simulink model "Power_Model_Official_Pars"  (R2023a)
settings: Solver=ode23t  StartTime=0.0  StopTime=1000  FixedStep=0.01  MaxStep=0.01  RelTol=1e-3  AbsTol=1e-3
values from neighbouring files (symbols this model uses):
  anode_tube_D = 0.01    [fuel_cell_battery_par.mat]
  cathode_tube_D = 0.05    [fuel_cell_battery_par.mat]
  comp_rpm_TLU = [0 1800 3600]    [fuel_cell_battery_par.mat]
  coolant_num_layers = 20    [fuel_cell_battery_par.mat]
  coolant_num_passes = 12    [fuel_cell_battery_par.mat]
  coolant_tube_D = 0.05    [fuel_cell_battery_par.mat]
  coolant_w_channels = 1    [fuel_cell_battery_par.mat]
  env_p = 0.101325    [fuel_cell_battery_par.mat]
  env_T = 20    [fuel_cell_battery_par.mat]
  env_yH20 = 0.0115436377169    [fuel_cell_battery_par.mat]
  env_yO2 = 0.21    [fuel_cell_battery_par.mat]
  radiator_air_area_fins = 11.5625    [fuel_cell_battery_par.mat]
  radiator_air_area_primary = 1.223125    [fuel_cell_battery_par.mat]
  radiator_eta_fin = 0.7    [fuel_cell_battery_par.mat]
  radiator_N_tubes = 25    [fuel_cell_battery_par.mat]
  radiator_rho = 2700    [fuel_cell_battery_par.mat]
  radiator_t_wall = 0.0001    [fuel_cell_battery_par.mat]
  radiator_tube_H = 0.0015    [fuel_cell_battery_par.mat]
  radiator_W = 0.025    [fuel_cell_battery_par.mat]
  stack_area = 280    [fuel_cell_battery_par.mat]
  stack_iL = 1.4    [fuel_cell_battery_par.mat]
  stack_mea_rho = 1800    [fuel_cell_battery_par.mat]
  stack_num_cells = 400    [fuel_cell_battery_par.mat]
  stack_num_channels = 8    [fuel_cell_battery_par.mat]
  stack_t_gdl = 250    [fuel_cell_battery_par.mat]
  stack_t_membrane = 125    [fuel_cell_battery_par.mat]
  stack_w_channels = 1    [fuel_cell_battery_par.mat]
undefined symbols (not defined in the file or in its folder): Bat, f_fc_auxpower, f_fc_currcmd_bpt, f_fc_h2flow, f_fc_heatflow, f_fc_tmpcmd_bpt, f_fc_voltage, Mot, N2_T
libraries: fl_lib x170, nesl_utility x78, FuelCell_lib x32, simulink x5, slpidlib x4, ee_lib x3, autolibshared x1, batteryecm_lib x1, simulink_extras x1
(part 1 of 9)
settings Model: Creator=Learning  LastModifiedBy=Leviathan
settings SolverCC: ZeroCrossAlgorithm=Adaptive
settings OptimizationCC: ReuseModelBlockBuffer=off
settings DebuggingCC: IgnoredZcDiagnostic=none
settings ModelReferenceCC: EnableRefExpFcnMdlSchedulingChecks=on
settings SimscapeCC: SimscapeLogType=all  SimscapeLogSimulationStatistics=on  SimscapeLogLimitData=off

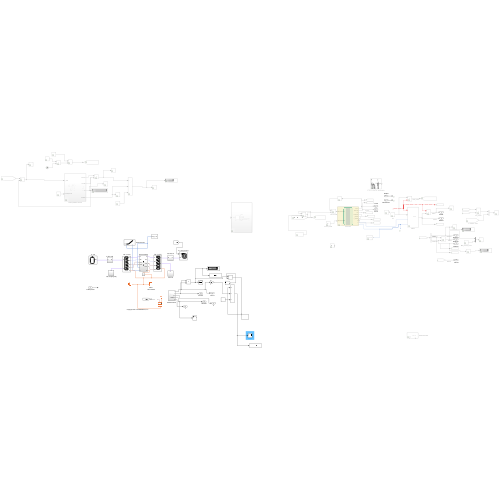
[thumbnail: Simulink's stored preview of the top-level diagram]
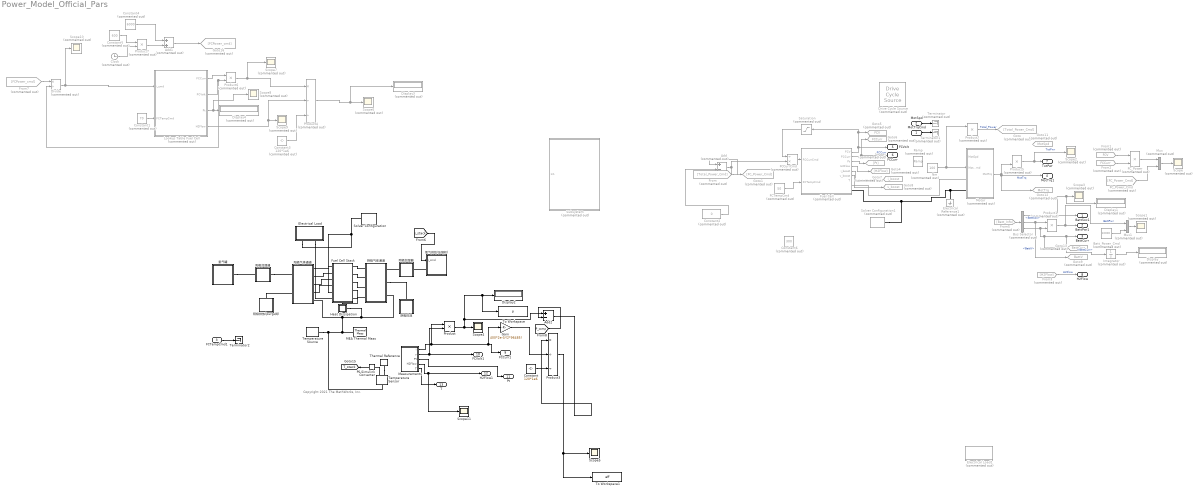
== system Power_Model_Official_Pars ==
  note: Copyright 2021 The MathWorks, Inc.
  MotTrqCmd : Inport
  MotSpd : Inport  Port=2
  FCTempCmd1 : Inport  Port=3
  Add : Sum  Commented=on  Inputs=+-
  Add1 : Sum  Commented=on
  Add2 : Sum  Inputs=+-
  Batt_Power_Cmd : Constant  Commented=on  Value=10000
  Bus Selector : BusSelector  Commented=on  OutputSignals=BattSoc,BattV,BattCurr
  Clock : Clock  Commented=on
  Constant : Constant  Value=120*1e6
  Constant1 : Constant  Commented=on  Value=70
  Constant2 : Constant  Commented=on  Value=0
  Constant3 : Constant  Commented=on  Value=120*1e6
  Constant4 : Constant  Commented=on  Value=6000
  Constant5 : Constant  Commented=on  Value=600
  Constant6 : Constant  Commented=on  Value=300
  Display{,1,3..4} (4 alike) : Display  Commented=on
  Display2 : Display
  Divide : Product  Commented=on  Inputs=*/
  Drive Cycle Source : autolibshared/Drive Cycle Source  Commented=on  cycleVar=FTP75  fileVar=L:\Bauto\matlab\test\toolbox\shared\autoblks\scenario\adac.txt  tfinal="2474  seconds"  cycleRepeat=off  outAccPort=off  outGearPort=off  gearList=No gear data  t_wot1=1  xdot_woto=0  xdot_wot1=26.8  t_wot2=30  xdot_wot2=0  t_wotend=40  srcUnit=m/s  outUnit=m/s  srcAccUnit=m/s/s  outAccUnit=m/s^2  dt=0  aMode=1  faultOption=off  velBnd=2  velBndUnit=mph  inUnit=m/s  timeBnd=1  failOption=off  stopSim=off  maxFaultCnt=10  maxFaultTime=2  maxTotFaultTime=15  traceOption=off  dtTrace=1  traceWindow=10  lastDCname=FTP75  lastOutUnit=mph  lastDT=0  lastTB=1  lastSB=2  forceCalcBound=off
  Electrical Load : Subsystem  Tag=PublishSubsystem  mask(Electrical Load){input_type=Ramp}
      mask prompts: input_type "Select one of the following scenarios:"
      settings: PortSchema="{\"entries\":[{\"content\":{\"sides\":[{\"content\":{},\"type\":\"ConnectorPlacement.EquallySpacedRectSide\",\"uuid\":\"cf26c57a-4aaa-4eca-a1cf-dab3379228b7\"},{\"content\":{\"side\":\"RIGHT\"},\"type\":\"ConnectorPlacement.EquallySpacedRectSide\",\"uuid\":\"bd4a28c6-f8d3-4492-9f61-a12eb17ccdd3\"},{\"content\":{\"side\":\"TOP\"},\"type\":\"ConnectorPlacement.EquallySpacedRectSide\",\"uuid\":\"7f54a4db-ccf4-4e3a-a135-4ada067d241f\"},{\"content\":{\"connectorIds\":[\"RConn1\",\"RConn2\"],\"side\":\"BOTTOM\"},\"type\":\"ConnectorPlacement.EquallySpacedRectSide\",\"uuid\":\"8817983d-3f79-43b3-9594-6d12f7dcf066\"}]},\"type\":\"ConnectorPlacement.EquallySpacedConnector\",\"uuid\":\"79253ea6-cd7f-4983-840a-f5cee3a4dd91\"}],\"packageUris\":[\"http://schema.mathworks.com/mf0/Connector/R2020b\"],\"version\":\"1.0\"}"
      mask TypeOptions input_type: Drive cycle | Ramp | Step
      mask Callback input_type:
      | activeVariant = get_param(gcb, 'input_type');
      | set_param([gcb '/Inputs'], 'OverrideUsingVariant', activeVariant)
      mask Display:
      | blk = get_param([gcb, '/Inputs'], 'CompiledActiveChoiceBlock');
      | eval(get_param(blk, 'MaskDisplay'))
  Electrical Load1 : Subsystem  Tag=PublishSubsystem  Commented=on  mask(Electrical Load){input_type=Ramp}
      mask prompts: input_type "Select one of the following scenarios:"
      settings: PortSchema="{\"entries\":[{\"content\":{\"sides\":[{\"content\":{},\"type\":\"ConnectorPlacement.EquallySpacedRectSide\",\"uuid\":\"cf26c57a-4aaa-4eca-a1cf-dab3379228b7\"},{\"content\":{\"side\":\"RIGHT\"},\"type\":\"ConnectorPlacement.EquallySpacedRectSide\",\"uuid\":\"bd4a28c6-f8d3-4492-9f61-a12eb17ccdd3\"},{\"content\":{\"side\":\"TOP\"},\"type\":\"ConnectorPlacement.EquallySpacedRectSide\",\"uuid\":\"7f54a4db-ccf4-4e3a-a135-4ada067d241f\"},{\"content\":{\"connectorIds\":[\"RConn1\",\"RConn2\"],\"side\":\"BOTTOM\"},\"type\":\"ConnectorPlacement.EquallySpacedRectSide\",\"uuid\":\"8817983d-3f79-43b3-9594-6d12f7dcf066\"}]},\"type\":\"ConnectorPlacement.EquallySpacedConnector\",\"uuid\":\"79253ea6-cd7f-4983-840a-f5cee3a4dd91\"}],\"packageUris\":[\"http://schema.mathworks.com/mf0/Connector/R2020b\"],\"version\":\"1.0\"}"
      mask TypeOptions input_type: Drive cycle | Ramp | Step
      mask Callback input_type:
      | activeVariant = get_param(gcb, 'input_type');
      | set_param([gcb '/Inputs'], 'OverrideUsingVariant', activeVariant)
      mask Display:
      | blk = get_param([gcb, '/Inputs'], 'CompiledActiveChoiceBlock');
      | eval(get_param(blk, 'MaskDisplay'))
  Electrical Reference1 : fl_lib/Electrical/Electrical Elements/Electrical Reference  Commented=on
  FCCurrCmd : Product  Commented=on  Inputs=/*
  FCTempCmd : Constant  Commented=on  Value=50
  FC_Power : Product  Commented=on
  FC_Power_Cmd : From  Commented=on  GotoTag=FC_Power_Cmd
  From : From  Commented=on  GotoTag=Total_Power_Cmd
  From1 : From  Commented=on  GotoTag=FCV  TagVisibility=global
  From2 : From  Commented=on  GotoTag=FCCurr  TagVisibility=global
  From3 : From  Commented=on  GotoTag=H2Flow
  From5 : From  Commented=on  GotoTag=Batt_Info
  From7 : From  Commented=on  GotoTag=FCPower_cmd
  Fuel Cell : Subsystem  Commented=on  VariantControl=0
      mask Display: image('fuel_cell_converter_IMAGE.png'); % Use "Edit Image" on toolstrip to change.
  Fuel Cell Stack : Subsystem  VariantControl=SSC
  Gain : Gain  Gain=400*2e-3/(2*96485)
  Goto : Goto  Commented=on  GotoTag=Total_Power_Cmd
  Goto1 : Goto  Commented=on  GotoTag=FC_Power_Cmd
  Goto11 : Goto  Commented=on  GotoTag=MotSpd  TagVisibility=global
  Goto12 : Goto  Commented=on  GotoTag=MotTrq  TagVisibility=global
  Goto13 : Goto  Commented=on  GotoTag=BattCurr  TagVisibility=global
  Goto16 : Goto  Commented=on  GotoTag=FCPower_cmd
  Goto2 : Goto  Commented=on  GotoTag=Pt
  Goto4 : Goto  Commented=on  GotoTag=H2Flow
  Goto5 : Goto  Commented=on  GotoTag=FCV  TagVisibility=global
  Goto6 : Goto  Commented=on  GotoTag=FCCurr  TagVisibility=global
  Goto7 : Goto  Commented=on  GotoTag=i_boost  TagVisibility=global
  Goto8 : Goto  Commented=on  GotoTag=v_boost  TagVisibility=global
  Goto9 : Goto  Commented=on  GotoTag=BattV  TagVisibility=global
  Heat Dissipation : Subsystem
      settings: PortSchema="{\"entries\":[{\"content\":{\"sides\":[{\"content\":{},\"type\":\"ConnectorPlacement.EquallySpacedRectSide\",\"uuid\":\"40b2385a-b20e-464f-8016-3228e4acac4a\"},{\"content\":{\"connectorIds\":[\"RConn1\"],\"side\":\"RIGHT\"},\"type\":\"ConnectorPlacement.EquallySpacedRectSide\",\"uuid\":\"0e95dc4b-d2da-4ab6-a6e9-e2cb275776ce\"},{\"content\":{\"connectorIds\":[\"LConn1\"],\"side\":\"TOP\"},\"type\":\"ConnectorPlacement.EquallySpacedRectSide\",\"uuid\":\"0f5995c7-26f6-433d-889b-dea78bcd2b2a\"},{\"content\":{\"side\":\"BOTTOM\"},\"type\":\"ConnectorPlacement.EquallySpacedRectSide\",\"uuid\":\"a2ee1c19-f9e9-4dbd-a9ff-92feea387e85\"}]},\"type\":\"ConnectorPlacement.EquallySpacedConnector\",\"uuid\":\"721753ea-9ada-4c74-8c6f-50b905d96904\"}],\"packageUris\":[\"http://schema.mathworks.com/mf0/Connector/R2020b\"],\"version\":\"1.0\"}"
  Integrator : Integrator  Commented=on
  Lookup Table Fuel Cell : Subsystem  Commented=on  VariantControl=Choice_3
      settings: PortSchema="{\"entries\":[{\"content\":{\"sides\":[{\"content\":{},\"type\":\"ConnectorPlacement.EquallySpacedRectSide\",\"uuid\":\"32248e1c-8adb-4301-a735-652c844f38d9\"},{\"content\":{\"side\":\"RIGHT\"},\"type\":\"ConnectorPlacement.EquallySpacedRectSide\",\"uuid\":\"e199895e-2a46-4791-8ec6-c72fbddb281a\"},{\"content\":{\"connectorIds\":[\"In1\",\"In2\"],\"side\":\"TOP\"},\"type\":\"ConnectorPlacement.EquallySpacedRectSide\",\"uuid\":\"d27f5cfc-8d50-4a08-b63d-60966cdd3a3e\"},{\"content\":{\"connectorIds\":[\"Out1\",\"Out2\",\"Out3\",\"Out4\"],\"side\":\"BOTTOM\"},\"type\":\"ConnectorPlacement.EquallySpacedRectSide\",\"uuid\":\"4de9f516-5cfd-4c93-92a2-161937995774\"}]},\"type\":\"ConnectorPlacement.EquallySpacedConnector\",\"uuid\":\"ebb74780-6fd4-4e24-9636-290cc1e1e603\"}],\"packageUris\":[\"http://schema.mathworks.com/mf0/Connector/R2020b\"],\"version\":\"1.0\"}"
  MEA Thermal Mass : fl_lib/Thermal/Thermal Elements/Thermal Mass  mass_type=foundation.enum.constant_variable.constant  mass=stack_mea_rho * stack_area*1e-4 * (stack_t_membrane + 2*stack_t_gdl)*1e-6 * stack_num_cells kg  sp_heat=stack_mea_cp J/kg/K  mass_min=1e-6 kg  num_ports=foundation.enum.numPorts2.one  m_specify=off  m_priority=High  m=1 kg  m_nominal_specify=off  m_nominal_unit=kg  m_nominal_value=1  T_specify=on  T_priority=High  T=env_T degC  T_nominal_specify=off  T_nominal_unit=K  T_nominal_value=1  Q_specify=off  Q_priority=None  Q=0 W  Q_nominal_specify=off  Q_nominal_unit=W  Q_nominal_value=1
  Measurements : Subsystem
  Motor : Subsystem  Commented=on
      mask Display: image('E:\Graduation Project File\Fuel_cell\Fuel_cell_model\Model_figure\emotor_simplified_IMAGE.png'); % 使用工具条上的 "编辑图像" 进行更改。
  Mux : Mux  Commented=on  Inputs=2
  Mux1 : Mux  Commented=on  Inputs=2
  Nm : Constant  Commented=on  Value=100
  PS-Simulink Converter : nesl_utility/PS-Simulink Converter  PhysicalDomain=network_engine_domain  SubClassName=ps_output  LeftPortType=input  RightPortType=output  PseudoPeriodic=off  Frequencies=[]  VectorFormat=1-D array  Unit=degC  AffineConversion=on
  Product : Product
  Product{1..2,5..7} (5 alike) : Product  Commented=on
  Product3 : Product  Inputs=*//
  Product4 : Product  Commented=on  Inputs=*//
  Ramp : simulink/Sources/Ramp  Commented=on  slope=1  start=0  InitialOutput=0
  Saturation : Saturate  Commented=on  UpperLimit=inf  LowerLimit=250
  Scope{,1..3,6..10} (9 alike) : Scope  Commented=on
  Scope11 : Scope
  Scope4 : Scope
  Scope5 : Scope
  Solver Configuration : nesl_utility/Solver Configuration  PhysicalDomain=network_engine_domain  SubClassName=solver  LeftPortType=input  RightPortType=generic  Tones=[]  Harmonics=[]  SimulateNoise=off  Profile=off  UseLocalSampling=off  EnableSwitchedLinearOptims=on  FrequencyDomain=off  UseCCode=off  RelTol=0.001  AbsTol=1e-06  MinStep=1e-09  ToWorkspace=off  RevertToSquareIcSolve=off  NumHomotopyIterations=100  PhasorMode=off  PhasorModeNumHarmonics=1  ConsistencySolver=NEWTON_XTOL_AFTER_FTOL  IndexReductionMethod=DerivativeReplacement  DoDC=off  ResidualTolerance=1e-09  ConsistencyTolSource=GLOBAL  ConsistencyAbsTol=0.001  ConsistencyRelTol=0.001  ConsistencyTolFactor=0.001  UseLocalSolver=off  LocalSolverChoice=NE_BACKWARD_EULER_ADVANCER  ResolveIndetEquations=on  FunctionEvalNumThread=1  LocalSolverSampleTime=0.001  DoFixedCost=off  MaxNonlinIter=3  MaxModeIter=2  ComputeImpulses=off  ImpulseIterations=2  LinearAlgebra=auto  LinearAlgebraNumThread=0  EquationFormulation=NE_TIME_EF  DelaysMemoryBudget=1024  AutomaticFiltering=on  FilteringTimeConstant=0.001  PartitionStorageMethod=AS_NEEDED  PartitionMemoryBudget=1024  PartitionMethod=ROBUST
  Solver Configuration1 : nesl_utility/Solver Configuration  Commented=on  PhysicalDomain=network_engine_domain  SubClassName=solver  LeftPortType=input  RightPortType=generic  Tones=[]  Harmonics=[]  SimulateNoise=off  Profile=off  UseLocalSampling=off  EnableSwitchedLinearOptims=on  FrequencyDomain=off  UseCCode=off  RelTol=0.001  AbsTol=1e-06  MinStep=1e-09  ToWorkspace=off  RevertToSquareIcSolve=off  NumHomotopyIterations=100  PhasorMode=off  PhasorModeNumHarmonics=1  ConsistencySolver=NEWTON_XTOL_AFTER_FTOL  IndexReductionMethod=DerivativeReplacement  DoDC=off  ResidualTolerance=1e-09  ConsistencyTolSource=GLOBAL  ConsistencyAbsTol=0.001  ConsistencyRelTol=0.001  ConsistencyTolFactor=0.001  UseLocalSolver=off  LocalSolverChoice=NE_BACKWARD_EULER_ADVANCER  ResolveIndetEquations=on  FunctionEvalNumThread=1  LocalSolverSampleTime=0.001  DoFixedCost=off  MaxNonlinIter=3  MaxModeIter=2  ComputeImpulses=off  ImpulseIterations=2  LinearAlgebra=auto  LinearAlgebraNumThread=0  EquationFormulation=NE_TIME_EF  DelaysMemoryBudget=1024  AutomaticFiltering=on  FilteringTimeConstant=0.001  PartitionStorageMethod=AS_NEEDED  PartitionMemoryBudget=1024  PartitionMethod=ROBUST
  Subsystem : Subsystem  Commented=on
  Temperature Sensor : fl_lib/Thermal/Thermal Sensors/Temperature Sensor  temperature_measure=foundation.enum.MeasurementReference.difference
  Temperature Source : fl_lib/Thermal/Thermal Sources/Temperature Source  temperature=70 degC
  Terminator : Terminator  Commented=on
  Terminator1 : Terminator  Commented=on
  Terminator2 : Terminator
  Thermal Reference : fl_lib/Thermal/Thermal Elements/Thermal Reference
  To Workspace : ToWorkspace  VariableName=p  SampleTime=1
  To Workspace1 : ToWorkspace  VariableName=eff  SampleTime=1
  氢气罐 : Subsystem  Tag=PublishSubsystem
      mask Display:
      | plot(0, 0)
      | plot(100, 100)
      | 
      | n = 20;
      | r = 20;
      | x1 = 15;
      | x2 = 65;
      | y1 = 5;
      | y2 = 85;
      | 
      | plot([x1 x1], [y1+r y2-r])
      | plot([x1+r x2-r], [y2 y2])
      | plot([x2 x2], [y2-r y1+r])
      | plot([x2-r x1+r], [y1 y1])
      | 
      | plot(cos(linspace(pi/2, pi, n))*r + x1+r, sin(linspace(pi/2, pi, n))*r + y2-r)
      | plot(cos(linspace(0, pi/2, n))*r + x2-r, sin(linspace(0, pi/2, n))*r + y2-r)
      | plot(cos(linspace(3*pi/2, 2*pi, n))*r + x2-r, sin(linspace(3*pi/2, 2*pi, n))*r + y1+r)
      | plot(cos(linspace(pi, 3*pi/2, n))*r + x1+r, sin(linspace(pi, 3*pi/2, n))*r + y1+r)
      | 
      | plot([-5 -5 5 5] + (x1+x2)/2, [0 5 5 0] + y2)
  氧气供给(压缩机) : Subsystem  Tag=PublishSubsystem
      mask Display:
      | plot(0, 0)
      | plot(100, 100)
      | 
      | n = 80;
      | r1 = 15;
      | r2 = 30;
      | 
      | plot(cos(linspace(0, 2*pi, n))*r1 + 65, sin(linspace(0, 2*pi, n))*r1 + 50)
      | plot(cos(linspace(0, 2*pi, n))*r2 + 65, sin(linspace(0, 2*pi, n))*r2 + 50)
      | 
      | plot([65 30 30 42], [80 80 70 70])
  阳极加湿器 : Subsystem  Tag=PublishSubsystem
  阳极排放(purge阀) : Subsystem  Tag=PublishSubsystem
      settings: PortSchema="{\"entries\":[{\"content\":{\"sides\":[{\"content\":{\"connectorIds\":[]},\"type\":\"ConnectorPlacement.EquallySpacedRectSide\",\"uuid\":\"6344d1cf-22ea-4a51-9588-07afca0fac15\"},{\"content\":{\"connectorIds\":[],\"side\":\"RIGHT\"},\"type\":\"ConnectorPlacement.EquallySpacedRectSide\",\"uuid\":\"a3908f81-9410-4056-87cd-9faba76d3fb8\"},{\"content\":{\"connectorIds\":[\"LConn1\"],\"side\":\"TOP\"},\"type\":\"ConnectorPlacement.EquallySpacedRectSide\",\"uuid\":\"a1c9e24d-adb9-4361-8e9b-feafccbbdb81\"}]},\"type\":\"ConnectorPlacement.EquallySpacedConnector\",\"uuid\":\"d5180d8f-18a0-491d-9fff-909db43c9aea\"}],\"packageUris\":[\"http://schema.mathworks.com/mf0/Connector/R2020b\"],\"version\":\"1.0\"}"
  阳极气体通道 : Subsystem  Tag=PublishSubsystem
      mask Display:
      | plot(0, 0)
      | plot(100, 100)
      | 
      | x1 = 25;
      | x2 = 65;
      | y1 = 23;
      | y2 = 95;
      | xt = 15;
      | yt = 9;
      | 
      | x_pattern = [x2 x2    x1+xt x1+xt   x1+xt   x2     ];
      | y_pattern = [y2 y2-yt y2-yt y2-2*yt y2-2*yt y2-2*yt];
      | 
      | plot([x1 x1 x2 x_pattern x_pattern      x_pattern      x_pattern         x2    x1], ...
      |      [y1-yt y2 y2 y_pattern y_pattern-2*yt y_pattern-4*yt y_pattern-6*yt y1-yt y1-yt])
  阴极加湿器 : Subsystem  Tag=PublishSubsystem
  阴极排放 : Subsystem  Tag=PublishSubsystem
      settings: PortSchema="{\"entries\":[{\"content\":{\"sides\":[{\"content\":{\"connectorIds\":[]},\"type\":\"ConnectorPlacement.EquallySpacedRectSide\",\"uuid\":\"6344d1cf-22ea-4a51-9588-07afca0fac15\"},{\"content\":{\"connectorIds\":[],\"side\":\"RIGHT\"},\"type\":\"ConnectorPlacement.EquallySpacedRectSide\",\"uuid\":\"a3908f81-9410-4056-87cd-9faba76d3fb8\"},{\"content\":{\"connectorIds\":[\"LConn1\"],\"side\":\"TOP\"},\"type\":\"ConnectorPlacement.EquallySpacedRectSide\",\"uuid\":\"a1c9e24d-adb9-4361-8e9b-feafccbbdb81\"}]},\"type\":\"ConnectorPlacement.EquallySpacedConnector\",\"uuid\":\"d5180d8f-18a0-491d-9fff-909db43c9aea\"}],\"packageUris\":[\"http://schema.mathworks.com/mf0/Connector/R2020b\"],\"version\":\"1.0\"}"
  阴极气体通道 : Subsystem  Tag=PublishSubsystem
      mask Display:
      | plot(0, 0)
      | plot(100, 100)
      | 
      | x1 = 35;
      | x2 = 75;
      | y1 = 23;
      | y2 = 95;
      | xt = 15;
      | yt = 9;
      | 
      | x_pattern = [x1 x1    x2-xt x2-xt   x2-xt   x1     ];
      | y_pattern = [y2 y2-yt y2-yt y2-2*yt y2-2*yt y2-2*yt];
      | 
      | plot([x2 x2 x1 x_pattern x_pattern      x_pattern      x_pattern         x1    x2], ...
      |      [y1-yt y2 y2 y_pattern y_pattern-2*yt y_pattern-4*yt y_pattern-6*yt y1-yt y1-yt])
  BattSoc1 : Outport  VectorParamsAs1DForOutWhenUnconnected=off
  BattPwr1 : Outport  Port=2  VectorParamsAs1DForOutWhenUnconnected=off
  BattCurr : Outport  Port=3  VectorParamsAs1DForOutWhenUnconnected=off
  MotTrq1 : Outport  Port=4  VectorParamsAs1DForOutWhenUnconnected=off
  FCVolt : Outport  Port=5  VectorParamsAs1DForOutWhenUnconnected=off
  FCCurr : Outport  Port=6  VectorParamsAs1DForOutWhenUnconnected=off
  TotPwr : Outport  Port=7
  H2Flow : Outport  Port=8  VectorParamsAs1DForOutWhenUnconnected=off
  FCCurr1 : Outport  Port=9
  FCVolt1 : Outport  Port=10
  Pt : Outport  Port=11
  H2Flow1 : Outport  Port=12
  T : Outport  Port=13
  tag scope: T_stack=global
  wires:
  Bus Selector/1 -> Display1/1, Scope3/1, BattSoc1/1  "<BattSoc>"
  FCTempCmd/1 -> Fuel Cell/2(FCTempCmd)
  Motor/1(MotTrq) -> Goto12/1, MotTrq1/1, Product5/2  "MotTrq"
  From3/1 -> H2Flow/1  "H2Flow"
  Product5/1 -> Scope2/1, TotPwr/1  "TotPwr"
  ? -> Product2/2, Product5/1, Goto11/1, Motor/1(MotSpd)
  Bus Selector/3 -> Goto13/1, Integrator/1, BattCurr/1, Product1/2  "<BattCurr>"
  Product1/1 -> Mux1/1, BattPwr1/1  "BattPwr"
  Fuel Cell/5(i_boost) -> Goto7/1
  From5/1 -> Bus Selector/1
  Nm/1 -> Product2/1, Motor/2(MotTrqCmd)
  Fuel Cell/2(FCCurr) -> Goto6/1, FCCurr/1  "FCCurr"
  Fuel Cell/3(Pt) -> Goto2/1
  Bus Selector/2 -> Product1/1, Goto9/1  "<BattV>"
  FCCurrCmd/1 -> Fuel Cell/1(FCCurrCmd)
  Saturation/1 -> FCCurrCmd/1
  MotSpd/1 -> Terminator/1
  MotTrqCmd/1 -> Terminator1/1
  Product2/1 -> Goto/1  "Total_Power"
  From/1 -> Add/1
  Constant2/1 -> Add/2
  Add/1 -> Goto1/1, FCCurrCmd/2
  From1/1 -> FC_Power/1
  From2/1 -> FC_Power/2
  Mux/1 -> Scope/1
  FC_Power/1 -> Mux/1
  FC_Power_Cmd/1 -> Mux/2
  Mux1/1 -> Scope1/1
  Batt_Power_Cmd/1 -> Mux1/2
  Fuel Cell/1(FCV) -> Saturation/1, Goto5/1, FCVolt/1
  Fuel Cell/4(H2Flow) -> Goto4/1
  Fuel Cell/6(v_boost) -> Goto8/1
  Integrator/1 -> Display/1
  Measurements/3(Pt) -> Pt/1
  Measurements/5(T) -> T/1
  FCTempCmd1/1 -> Terminator2/1
  PS-Simulink Converter/1 -> [T_stack]
  Measurements/4(H2Flow) -> Scope11/1, H2Flow1/1
  Measurements/1(i) -> Product/1, Gain/1, FCCurr1/1
  Measurements/2(v) -> Product/2, FCVolt1/1
  Product/1 -> Add2/1, To Workspace/1, Display2/1, Scope4/1
  [i_stack] -> 氧气供给(压缩机)/1(i_cmd)
  Constant/1 -> Product3/3
  Product3/1 -> To Workspace1/1, Scope5/1
  Constant1/1 -> Lookup Table Fuel Cell/2(FCTempCmd)
  Lookup Table Fuel Cell/4(H2Flow) -> Product4/2, Scope9/1
  Product4/1 -> Display3/1, Scope6/1
  Constant3/1 -> Product4/3
  Product6/1 -> Scope7/1, Product4/1
  Lookup Table Fuel Cell/1(FCCurr) -> Product6/1
  Lookup Table Fuel Cell/2(FCVolt) -> Divide/2, Product6/2
  From7/1 -> Divide/1
  Clock/1 -> Product7/2
  Constant5/1 -> Product7/1
  Product7/1 -> Add1/2
  Constant4/1 -> Add1/1
  Add1/1 -> Goto16/1
  Lookup Table Fuel Cell/3(Pt) -> Scope8/1, Display4/1
  Divide/1 -> Lookup Table Fuel Cell/1(i_cmd), Scope10/1
  Gain/1 -> Product3/2
  [P_comp] -> Add2/2
  Add2/1 -> Product3/1
  connections:
  Electrical Reference1/LConn1 -- Motor/LConn2 -- Solver Configuration1/RConn1 -- Fuel Cell/RConn2
  Motor/LConn1 -- Fuel Cell/RConn1
  Heat Dissipation/RConn1 -- MEA Thermal Mass/LConn1 -- Temperature Sensor/LConn1 -- Temperature Source/LConn1 -- 阳极气体通道/RConn5 -- 阴极气体通道/RConn3
  阳极加湿器/RConn1 -- 阳极气体通道/LConn1
  Fuel Cell Stack/RConn1 -- 阴极气体通道/LConn1
  Fuel Cell Stack/RConn3 -- 阴极气体通道/LConn3
  氢气罐/RConn1 -- 阳极加湿器/LConn1
  Fuel Cell Stack/RConn2 -- 阴极气体通道/LConn2
  Fuel Cell Stack/LConn4 -- 阳极气体通道/RConn4
  Fuel Cell Stack/LConn1 -- 阳极气体通道/RConn1
  阳极排放(purge阀)/LConn1 -- 阳极气体通道/LConn2
  氧气供给(压缩机)/LConn1 -- 阴极加湿器/RConn1
  Fuel Cell Stack/LConn3 -- 阳极气体通道/RConn3
  Fuel Cell Stack/RConn5 -- Heat Dissipation/LConn1
  阴极气体通道/RConn2 -- 阴极排放/LConn1
  Fuel Cell Stack/LConn2 -- 阳极气体通道/RConn2
  阴极加湿器/LConn1 -- 阴极气体通道/RConn1
  Thermal Reference/LConn1 -- Temperature Sensor/RConn1
  PS-Simulink Converter/LConn1 -- Temperature Sensor/RConn2
  Fuel Cell Stack/RConn4 -- 阴极气体通道/LConn4
  Electrical Load/RConn1 -- Solver Configuration/RConn1 -- Fuel Cell Stack/LConn5
  Electrical Load/RConn2 -- Fuel Cell Stack/LConn6

== system Power_Model_Official_Pars/Electrical Load ==
  Controlled Current Source : fl_lib/Electrical/Electrical Sources/Controlled Current Source
  Electrical Reference : fl_lib/Electrical/Electrical Elements/Electrical Reference
  Inputs : Subsystem  Variant=on  VariantControlMode=label  LabelModeActiveChoice=Ramp
      settings: PortSchema="{\"entries\":[{\"content\":{\"sides\":[{\"content\":{\"connectorIds\":[\"LConn1\"]},\"type\":\"ConnectorPlacement.EquallySpacedRectSide\",\"uuid\":\"316ab41f-9548-4c29-941b-82cd3006a9cc\"},{\"content\":{\"side\":\"RIGHT\"},\"type\":\"ConnectorPlacement.EquallySpacedRectSide\",\"uuid\":\"21ddf6a1-5f8a-47a4-ab15-3c27c3a556ce\"},{\"content\":{\"connectorIds\":[\"LConn2\"],\"side\":\"TOP\"},\"type\":\"ConnectorPlacement.EquallySpacedRectSide\",\"uuid\":\"59191a52-f145-4ac2-9cf2-0e0b54b3d2a8\"}]},\"type\":\"ConnectorPlacement.EquallySpacedConnector\",\"uuid\":\"e8f988fd-b412-4b1a-aaea-374cf82170cc\"}],\"packageUris\":[\"http://schema.mathworks.com/mf0/Connector/R2020b\"],\"version\":\"1.0\"}"
      mask Display:
      | blk = get_param(gcb, 'CompiledActiveChoiceBlock');
      | eval(get_param(blk, 'MaskDisplay'))
  Voltage Sensor : fl_lib/Electrical/Electrical Sensors/Voltage Sensor
  - : PMIOPort  Side=Right
  + : PMIOPort  Port=2  Side=Right
  connections:
  Electrical Reference/LConn1 -- Controlled Current Source/LConn1 -- -/RConn1 -- Voltage Sensor/RConn2
  +/RConn1 -- Voltage Sensor/LConn1 -- Controlled Current Source/RConn2
  Inputs/LConn1 -- Controlled Current Source/RConn1
  Voltage Sensor/RConn1 -- Inputs/LConn2

== system Power_Model_Official_Pars/Electrical Load1 ==
  Controlled Current Source : fl_lib/Electrical/Electrical Sources/Controlled Current Source
  Electrical Reference : fl_lib/Electrical/Electrical Elements/Electrical Reference
  Inputs : Subsystem  Variant=on  VariantControlMode=label  LabelModeActiveChoice=Ramp
      settings: PortSchema="{\"entries\":[{\"content\":{\"sides\":[{\"content\":{\"connectorIds\":[\"LConn1\"]},\"type\":\"ConnectorPlacement.EquallySpacedRectSide\",\"uuid\":\"316ab41f-9548-4c29-941b-82cd3006a9cc\"},{\"content\":{\"side\":\"RIGHT\"},\"type\":\"ConnectorPlacement.EquallySpacedRectSide\",\"uuid\":\"21ddf6a1-5f8a-47a4-ab15-3c27c3a556ce\"},{\"content\":{\"connectorIds\":[\"LConn2\"],\"side\":\"TOP\"},\"type\":\"ConnectorPlacement.EquallySpacedRectSide\",\"uuid\":\"59191a52-f145-4ac2-9cf2-0e0b54b3d2a8\"}]},\"type\":\"ConnectorPlacement.EquallySpacedConnector\",\"uuid\":\"e8f988fd-b412-4b1a-aaea-374cf82170cc\"}],\"packageUris\":[\"http://schema.mathworks.com/mf0/Connector/R2020b\"],\"version\":\"1.0\"}"
      mask Display:
      | blk = get_param(gcb, 'CompiledActiveChoiceBlock');
      | eval(get_param(blk, 'MaskDisplay'))
  Voltage Sensor : fl_lib/Electrical/Electrical Sensors/Voltage Sensor
  - : PMIOPort  Side=Right
  + : PMIOPort  Port=2  Side=Right
  connections:
  Electrical Reference/LConn1 -- Controlled Current Source/LConn1 -- -/RConn1 -- Voltage Sensor/RConn2
  +/RConn1 -- Voltage Sensor/LConn1 -- Controlled Current Source/RConn2
  Inputs/LConn1 -- Controlled Current Source/RConn1
  Voltage Sensor/RConn1 -- Inputs/LConn2

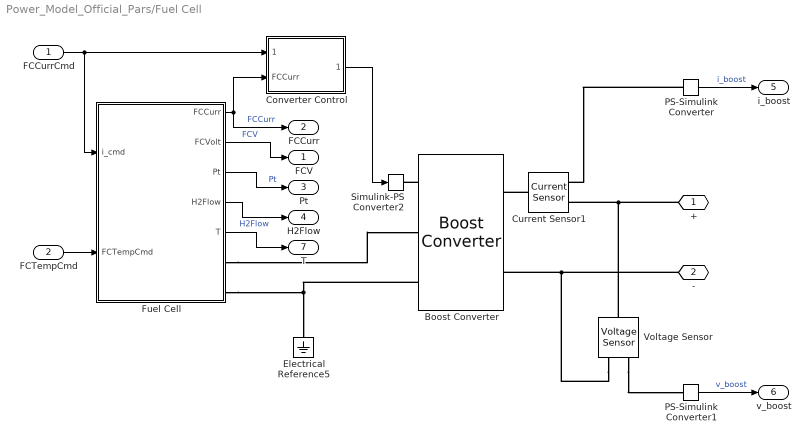
== system Power_Model_Official_Pars/Fuel Cell ==
  FCCurrCmd : Inport
  FCTempCmd : Inport  Port=2
  Boost Converter : ee_lib/Semiconductors & Converters/Converters/Boost Converter  port_option=ee.enum.controlport.ps  device_type=ee.enum.converters.switchingdevice.averaged  Vf=0.8 V  Ron=FCDCDC.avgSwitchResistance Ohm  Rds=0.001 Ohm  Goff=1e-5 1/Ohm  Vgt=1 V  Vgt_off=-1 V  Ih=1 A  Vth=6 V  K=0  diode_param=ee.enum.converters.diode.nodynamics  diode_Vf=FCDCDC.diodeFwdVolt V  diode_Ron=FCDCDC.diodeOnResistance Ohm  diode_Goff=FCDCDC.diodeOffConductance 1/Ohm  diode_C=50 nF  diode_iRM=-235 A  diode_iF=300 A  diode_idot=-50 A/us  diode_trr_param=ee.enum.converters.diodetrr.trr_factor  diode_trr_factor=3  diode_trr=15 us  diode_Qrr=1500 s*uA  Lf=FCDCDC.inductance H  Rl=FCDCDC.inductorSeriesResistance Ohm  Cf=FCDCDC.capacitance F  Rf=FCDCDC.CapEffSeriesResistance Ohm  snubber_type=ee.enum.converters.snubber.exclude  Cs=1e-7 F  Rs=0.1 Ohm  iL_specify=on  iL_priority=High  iL=0 A  iL_nominal_specify=off  iL_nominal_unit=A  iL_nominal_value=1  vc_specify=on  vc_priority=High  vc=FCDCDC.Vout V  vc_nominal_specify=off  vc_nominal_unit=V  vc_nominal_value=1
      settings: InternalSimscapePortConfiguration="{\"Bottom\":[],\"Left\":[{\"id\":\"G\",\"label\":\"G\",\"type\":\"input\"},{\"id\":\"p1\",\"label\":\"1+\",\"type\":\"foundation.electrical.electrical\"},{\"id\":\"n1\",\"label\":\"1-\",\"type\":\"foundation.electrical.electrical\"}],\"Right\":[{\"id\":\"p2\",\"label\":\"2+\",\"type\":\"foundation.electrical.electrical\"},{\"id\":\"n2\",\"label\":\"2-\",\"type\":\"foundation.electrical.electrical\"}],\"Top\":[]}"
  Converter Control : Subsystem
  Current Sensor1 : fl_lib/Electrical/Electrical Sensors/Current Sensor
  Electrical Reference5 : fl_lib/Electrical/Electrical Elements/Electrical Reference
  Fuel Cell : Subsystem  Variant=on  VariantControlMode=label  VariantControl=Choice  LabelModeActiveChoice=Choice_1
  PS-Simulink Converter : nesl_utility/PS-Simulink Converter  PhysicalDomain=network_engine_domain  SubClassName=ps_output  LeftPortType=input  RightPortType=output  PseudoPeriodic=off  Frequencies=[]  VectorFormat=inherit  Unit=inherit  AffineConversion=off
  PS-Simulink Converter1 : nesl_utility/PS-Simulink Converter  PhysicalDomain=network_engine_domain  SubClassName=ps_output  LeftPortType=input  RightPortType=output  PseudoPeriodic=off  Frequencies=[]  VectorFormat=inherit  Unit=inherit  AffineConversion=off
  Simulink-PS Converter2 : nesl_utility/Simulink-PS Converter  PhysicalDomain=network_engine_domain  SubClassName=ps_input  LeftPortType=input  RightPortType=output  PseudoPeriodic=off  Frequencies=[]  NoiseDistribution=none  NoiseParameters=[]  Unit=1  AffineConversion=off  FilteringAndDerivatives=provide  SimscapeFilterOrder=1  InputFilterTimeConstant=0.001  UdotUserProvided=0
  Voltage Sensor : fl_lib/Electrical/Electrical Sensors/Voltage Sensor
  + : PMIOPort  Side=Right
  - : PMIOPort  Port=2  Side=Right
  FCV : Outport
  FCCurr : Outport  Port=2
  Pt : Outport  Port=3
  H2Flow : Outport  Port=4
  i_boost : Outport  Port=5
  v_boost : Outport  Port=6
  T : Outport  Port=7
  wires:
  Converter Control/1(u_boost) -> Simulink-PS Converter2/1
  Fuel Cell/1(FCCurr) -> FCCurr/1, Converter Control/2(FCCurr)  "FCCurr"
  FCCurrCmd/1 -> Fuel Cell/1(i_cmd), Converter Control/1(FCCurrCmd)
  FCTempCmd/1 -> Fuel Cell/2(FCTempCmd)
  Fuel Cell/2(FCVolt) -> FCV/1  "FCV"
  Fuel Cell/3(Pt) -> Pt/1  "Pt"
  Fuel Cell/4(H2Flow) -> H2Flow/1  "H2Flow"
  PS-Simulink Converter/1 -> i_boost/1  "i_boost"
  PS-Simulink Converter1/1 -> v_boost/1  "v_boost"
  Fuel Cell/5(T) -> T/1
  connections:
  Boost Converter/LConn1 -- Simulink-PS Converter2/RConn1
  -/RConn1 -- Voltage Sensor/RConn2 -- Boost Converter/RConn2
  +/RConn1 -- Voltage Sensor/LConn1 -- Current Sensor1/RConn2
  Current Sensor1/LConn1 -- Boost Converter/RConn1
  Boost Converter/LConn3 -- Fuel Cell/RConn2 -- Electrical Reference5/LConn1
  PS-Simulink Converter/LConn1 -- Current Sensor1/RConn1
  Fuel Cell/RConn1 -- Boost Converter/LConn2
  Voltage Sensor/RConn1 -- PS-Simulink Converter1/LConn1

== system Power_Model_Official_Pars/Fuel Cell Stack ==
  Membrane Electrode Assembly : SimscapeComponentBlock  SourceFile=FuelCell  ComponentPath=FuelCell  ComponentVariants="[\"FuelCell\"]"  ComponentVariantNames="[\"FuelCell\"]"  ClassName=FuelCell  SchemaVersion=1  N_cell=stack_num_cells  area_cell=stack_area cm^2  t_membrane=stack_t_membrane um  t_gdl_A=stack_t_gdl um  t_gdl_C=stack_t_gdl um  io=stack_io A/cm^2  iL=stack_iL A/cm^2  alpha=0.28  D_H2O_gdl_A=0.07 cm^2/s  D_H2O_gdl_C=0.07 cm^2/s  rho_membrane=2000 kg/m^3  M_membrane=1.1 kg/mol  i_specify=off  i_priority=None  i=0 A  i_nominal_specify=off  i_nominal_unit=A  i_nominal_value=1  Q_specify=off  Q_priority=None  Q=0 W  Q_nominal_specify=off  Q_nominal_unit=W  Q_nominal_value=1  a_H2O_acl_specify=off  a_H2O_acl_priority=None  a_H2O_acl=0.5  a_H2O_acl_nominal_specify=off  a_H2O_acl_nominal_unit=1  a_H2O_acl_nominal_value=1  a_H2O_ccl_specify=off  a_H2O_ccl_priority=None  a_H2O_ccl=0.5  a_H2O_ccl_nominal_specify=off  a_H2O_ccl_nominal_unit=1  a_H2O_ccl_nominal_value=1
      settings: CopyFcn=simscape.engine.sli.internal.componentblockcallback(gcbh,'COPY')  PreCopyFcn=simscape.engine.sli.internal.componentblockcallback(gcbh,'PRECOPY')  PreDeleteFcn=simscape.engine.sli.internal.componentblockcallback(gcbh,'PREDELETE')  InternalSimscapePortConfiguration="{\"Bottom\":[{\"id\":\"H\",\"label\":\"H\",\"type\":\"foundation.thermal.thermal\"}],\"Left\":[{\"id\":\"A\",\"label\":\"A\",\"type\":\"foundation.moist_air.moist_air\"},{\"id\":\"SA\",\"label\":\"SA\",\"type\":\"foundation.moist_air.moist_air_source\"},{\"id\":\"FAi\",\"label\":\"FAi\",\"type\":\"input\"},{\"id\":\"FAo\",\"label\":\"FAo\",\"type\":\"input\"}],\"Right\":[{\"id\":\"C\",\"label\":\"C\",\"type\":\"foundation.moist_air.moist_air\"},{\"id\":\"SC\",\"label\":\"SC\",\"type\":\"foundation.moist_air.moist_air_source\"},{\"id\":\"FCi\",\"label\":\"FCi\",\"type\":\"input\"},{\"id\":\"FCo\",\"label\":\"FCo\",\"type\":\"input\"}],\"Top\":[{\"id\":\"n\",\"label\":\"-\",\"type\":\"foundation.electrical.electrical\"},{\"id\":\"p\",\"label\":\"+\",\"type\":\"foundation.electrical.electrical\"}]}"
      mask Type: Fuel Cell
  A : PMIOPort  Side=Left
  SA : PMIOPort  Port=2  Side=Left
  FAi : PMIOPort  Port=3  Side=Left
  FAo : PMIOPort  Port=4  Side=Left
  - : PMIOPort  Port=5  Side=Left
  + : PMIOPort  Port=6  Side=Left
  C : PMIOPort  Port=7  Side=Right
  SC : PMIOPort  Port=8  Side=Right
  FCi : PMIOPort  Port=9  Side=Right
  FCo : PMIOPort  Port=10  Side=Right
  H : PMIOPort  Port=11  Side=Right
  connections:
  Membrane Electrode Assembly/LConn4 -- FAo/RConn1
  Membrane Electrode Assembly/LConn3 -- FAi/RConn1
  Membrane Electrode Assembly/RConn5 -- H/RConn1
  Membrane Electrode Assembly/LConn5 -- -/RConn1
  Membrane Electrode Assembly/LConn6 -- +/RConn1
  Membrane Electrode Assembly/RConn1 -- C/RConn1
  Membrane Electrode Assembly/RConn4 -- FCo/RConn1
  Membrane Electrode Assembly/RConn3 -- FCi/RConn1
  Membrane Electrode Assembly/RConn2 -- SC/RConn1
  Membrane Electrode Assembly/LConn1 -- A/RConn1
  Membrane Electrode Assembly/LConn2 -- SA/RConn1

== system Power_Model_Official_Pars/Heat Dissipation ==
  Heat Flow Rate Sensor : fl_lib/Thermal/Thermal Sensors/Heat Flow Rate Sensor
  PS-Simulink Converter : nesl_utility/PS-Simulink Converter  PhysicalDomain=network_engine_domain  SubClassName=ps_output  LeftPortType=input  RightPortType=output  PseudoPeriodic=off  Frequencies=[]  VectorFormat=1-D array  Unit=kW  AffineConversion=off
  A : PMIOPort  Side=Left
  B : PMIOPort  Port=2  Side=Right
  tag scope: Q_stack=global
  wires:
  PS-Simulink Converter/1 -> [Q_stack]
  connections:
  Heat Flow Rate Sensor/RConn1 -- PS-Simulink Converter/LConn1
  B/RConn1 -- Heat Flow Rate Sensor/RConn2
  A/RConn1 -- Heat Flow Rate Sensor/LConn1

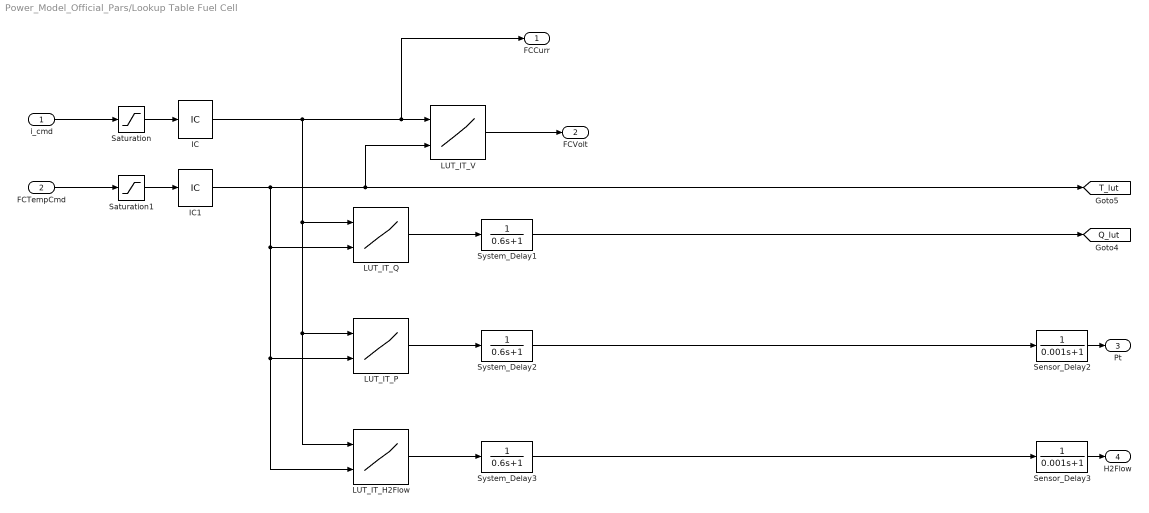
== system Power_Model_Official_Pars/Lookup Table Fuel Cell ==
  i_cmd : Inport
  FCTempCmd : Inport  Port=2
  IC : InitialCondition  Value=f_fc_currcmd_bpt(1)
  IC1 : InitialCondition  Value=f_fc_tmpcmd_bpt(1)
  LUT_IT_H2Flow : Lookup_n-D  BreakpointsForDimension1=f_fc_currcmd_bpt  BreakpointsForDimension2=f_fc_tmpcmd_bpt  Table=f_fc_h2flow  InterpMethod=Linear Lagrange  InternalRulePriority=Speed  RndMeth=Simplest
      settings: InputPortMap=u0,u1
  LUT_IT_P : Lookup_n-D  BreakpointsForDimension1=f_fc_currcmd_bpt  BreakpointsForDimension2=f_fc_tmpcmd_bpt  Table=f_fc_auxpower  InternalRulePriority=Speed  RndMeth=Simplest
      settings: InputPortMap=u0,u1
  LUT_IT_Q : Lookup_n-D  BreakpointsForDimension1=f_fc_currcmd_bpt  BreakpointsForDimension2=f_fc_tmpcmd_bpt  Table=f_fc_heatflow  InternalRulePriority=Speed  RndMeth=Simplest
      settings: InputPortMap=u0,u1
  LUT_IT_V : Lookup_n-D  BreakpointsForDimension1=f_fc_currcmd_bpt  BreakpointsForDimension2=f_fc_tmpcmd_bpt  Table=f_fc_voltage  InternalRulePriority=Speed  RndMeth=Simplest
      settings: InputPortMap=u0,u1
  Saturation : Saturate  UpperLimit=max(f_fc_currcmd_bpt)  LowerLimit=0
  Saturation1 : Saturate  UpperLimit=max(f_fc_tmpcmd_bpt)  LowerLimit=0
  Sensor_Delay2 : TransferFcn  Denominator=[0.001 1]
  Sensor_Delay3 : TransferFcn  Denominator=[0.001 1]
  System_Delay1 : TransferFcn  Denominator=[0.6 1]
  System_Delay2 : TransferFcn  Denominator=[0.6 1]
  System_Delay3 : TransferFcn  Denominator=[0.6 1]
  FCCurr : Outport
  FCVolt : Outport  Port=2
  Pt : Outport  Port=3
  H2Flow : Outport  Port=4
  tag scope: Q_lut=global, T_lut=global
  wires:
  IC/1 -> LUT_IT_H2Flow/1, LUT_IT_P/1, LUT_IT_Q/1, FCCurr/1, LUT_IT_V/1
  LUT_IT_V/1 -> FCVolt/1
  System_Delay2/1 -> Sensor_Delay2/1
  Sensor_Delay2/1 -> Pt/1
  Sensor_Delay3/1 -> H2Flow/1
  System_Delay3/1 -> Sensor_Delay3/1
  Saturation/1 -> IC/1
  Saturation1/1 -> IC1/1
  i_cmd/1 -> Saturation/1
  FCTempCmd/1 -> Saturation1/1
  LUT_IT_H2Flow/1 -> System_Delay3/1
  LUT_IT_P/1 -> System_Delay2/1
  IC1/1 -> LUT_IT_V/2, [T_lut], LUT_IT_H2Flow/2, LUT_IT_P/2, LUT_IT_Q/2
  LUT_IT_Q/1 -> System_Delay1/1
  System_Delay1/1 -> [Q_lut]

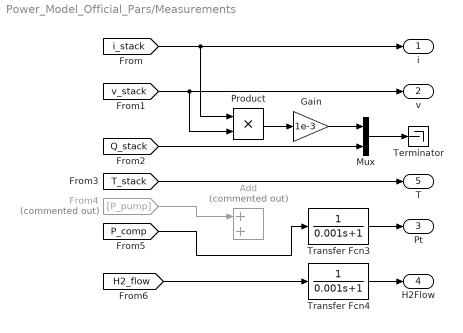
== system Power_Model_Official_Pars/Measurements ==
  Add : Sum  Commented=on
  From4 : From  Commented=on  GotoTag=P_pump
  Gain : Gain  Gain=1e-3
  Mux : Mux  Inputs=2
  Product : Product
  Terminator : Terminator
  Transfer Fcn3 : TransferFcn  Denominator=[0.001 1]
  Transfer Fcn4 : TransferFcn  Denominator=[0.001 1]
  i : Outport
  v : Outport  Port=2
  Pt : Outport  Port=3
  H2Flow : Outport  Port=4
  T : Outport  Port=5
  wires:
  Gain/1 -> Mux/1
  Mux/1 -> Terminator/1
  Product/1 -> Gain/1
  [Q_stack] -> Mux/2
  [T_stack] -> T/1
  [i_stack] -> i/1, Product/1
  [v_stack] -> v/1, Product/2
  From4/1 -> Add/1
  Transfer Fcn3/1 -> Pt/1
  [H2_flow] -> Transfer Fcn4/1
  Transfer Fcn4/1 -> H2Flow/1
  [P_comp] -> Transfer Fcn3/1

== system Power_Model_Official_Pars/Motor ==
  MotSpd : Inport
  MotTrqCmd : Inport  Port=2
  Elec Sensor : Subsystem
  Mechanical Rotational Reference1 : fl_lib/Mechanical/Rotational Elements/Mechanical Rotational Reference
  Motor : ee_lib/Electromechanical/Motor & Drive (System Level)  torque_speed_param=ee.enum.electromech.envelope.tabulated  overtorque_param=ee.enum.electromech.overtorque.no  T_t=Mot.maxT N*m  T_t_intermittent=[.36, .32, .28, 0] N*m  T_t_2D=[.09, .09, .09; .08, .08, .08; .07, .07, .07; 0, 0, 0] N*m  T_t_intermittent_2D=[.36, .36, .36; .32, .32, .32; .28, .28, .28; 0, 0, 0] N*m  w_t=Mot.w_eff_bp rpm  vdc_t=[6, 12, 24] V  torque_max=0.1 N*m  power_max=30 W  torque_max_intermittent=0.4 N*m  power_max_intermittent=120 W  time_overtorque=30 s  time_recover=60 s  Tc=Mot.Tc_Mot s  losses_param=3  eff=100  w_eff=3750 rpm  T_eff=0.08 N*m  Piron=0 W  Pbase=0 W  w_eff_vec=Mot.w_eff_bp rpm  T_eff_vec=Mot.T_eff_bp N*m  v_eff_vec=[100, 250, 400] V  losses_mat=[1.49, 1.67, 2.21, 3.1; .42, .69, 1.14, 2.03; .06, .24, .78, 1.68; .42, .69, 1.14, 2.03; 1.49, 1.67, 2.21, 3.1] W  efficiency_mat=Mot.efficiency_table  losses_mat_3D=ones(5, 4, 3) W  efficiency_mat_3D=95 * ones(5, 4, 3)  Res=Mot.supplyRes Ohm  enable_fault=simscape.enum.onoff.off  fault_condition=1  fault_threshold=0.5  J=Mot.inertia kg*m^2  lam=Mot.damping N*m/(rad/s)  speed0=0 rpm  faulted_specify=off  faulted_priority=None  faulted=0  faulted_nominal_specify=off  faulted_nominal_unit=1  faulted_nominal_value=1  torqueLimitContinuous_specify=off  torqueLimitContinuous_priority=None  torqueLimitContinuous=0 N*m  torqueLimitContinuous_nominal_specify=off  torqueLimitContinuous_nominal_unit=N*m  torqueLimitContinuous_nominal_value=1  alpha=3.93e-3 1/K  Tmeas=25 degC  Tmeas2=125 degC  losses_mat_T2=[1.49, 1.74, 2.49, 3.74; .42, .67, 1.42, 2.67; .06, .31, 1.06, 2.31; .42, .67, 1.42, 2.67; 1.49, 1.74, 2.49, 3.74] W  efficiency_mat_T2=[95, 95, 95, 95; 95, 95, 95, 95; 95, 95, 95, 95; 95, 95, 95, 95; 95, 95, 95, 95]  losses_mat_3D_T2=ones(5, 4, 3) W  efficiency_mat_3D_T2=95 * ones(5, 4, 3)  thermal_mass=100 J/K  initial_temperature=25 degC
  Simulink Interface : Subsystem
      settings: PortSchema="{\"entries\":[{\"content\":{\"sides\":[{\"content\":{\"connectorIds\":[\"In1\"]},\"type\":\"ConnectorPlacement.EquallySpacedRectSide\",\"uuid\":\"bf4125d2-d804-43ee-b309-19af55b24a20\"},{\"content\":{\"connectorIds\":[\"Out1\"],\"side\":\"RIGHT\"},\"type\":\"ConnectorPlacement.EquallySpacedRectSide\",\"uuid\":\"b387e632-ddea-4493-9ae8-5e997efec9a6\"},{\"content\":{\"connectorIds\":[\"LConn1\",\"LConn2\"],\"side\":\"TOP\"},\"type\":\"ConnectorPlacement.EquallySpacedRectSide\",\"uuid\":\"41fd5ea6-0488-466e-8be0-697a42498d14\"}]},\"type\":\"ConnectorPlacement.EquallySpacedConnector\",\"uuid\":\"25cf6a75-933f-4ef5-8c77-b93f7c2ffe1f\"}],\"packageUris\":[\"http://schema.mathworks.com/mf0/Connector/R2020b\"],\"version\":\"1.0\"}"
  Simulink-PS Converter3 : nesl_utility/Simulink-PS Converter  PhysicalDomain=network_engine_domain  SubClassName=ps_input  LeftPortType=input  RightPortType=output  PseudoPeriodic=off  Frequencies=[]  NoiseDistribution=none  NoiseParameters=[]  Unit=N*m  AffineConversion=off  FilteringAndDerivatives=provide  SimscapeFilterOrder=1  InputFilterTimeConstant=0.001  UdotUserProvided=0
  + : PMIOPort  Side=Left
  - : PMIOPort  Port=2  Side=Left
  MotTrq : Outport  VectorParamsAs1DForOutWhenUnconnected=off
  wires:
  MotTrqCmd/1 -> Simulink-PS Converter3/1
  MotSpd/1 -> Simulink Interface/1(MotSpd)
  Simulink Interface/1(MotTrq) -> MotTrq/1
  connections:
  -/RConn1 -- Motor/RConn1
  Simulink Interface/LConn1 -- Mechanical Rotational Reference1/LConn1 -- Motor/RConn3
  Motor/LConn2 -- Simulink-PS Converter3/RConn1
  Motor/LConn3 -- Simulink Interface/LConn2
  +/RConn1 -- Elec Sensor/LConn1
  Elec Sensor/RConn1 -- Motor/LConn1

== system Power_Model_Official_Pars/Subsystem ==
  In1 : Inport
  Battery System : Subsystem  VariantControl=0
      mask Display: image('E:\Graduation Project File\Fuel_cell\Fuel_cell_model\Model_figure\battery_system_IMAGE.png'); % 使用工具条上的 "编辑图像" 进行更改。
  Electrical Load9 : Subsystem  Tag=PublishSubsystem  mask(Electrical Load){input_type=Ramp}
      mask prompts: input_type "Select one of the following scenarios:"
      settings: PortSchema="{\"entries\":[{\"content\":{\"sides\":[{\"content\":{},\"type\":\"ConnectorPlacement.EquallySpacedRectSide\",\"uuid\":\"cf26c57a-4aaa-4eca-a1cf-dab3379228b7\"},{\"content\":{\"side\":\"RIGHT\"},\"type\":\"ConnectorPlacement.EquallySpacedRectSide\",\"uuid\":\"bd4a28c6-f8d3-4492-9f61-a12eb17ccdd3\"},{\"content\":{\"side\":\"TOP\"},\"type\":\"ConnectorPlacement.EquallySpacedRectSide\",\"uuid\":\"7f54a4db-ccf4-4e3a-a135-4ada067d241f\"},{\"content\":{\"connectorIds\":[\"RConn1\",\"RConn2\"],\"side\":\"BOTTOM\"},\"type\":\"ConnectorPlacement.EquallySpacedRectSide\",\"uuid\":\"8817983d-3f79-43b3-9594-6d12f7dcf066\"}]},\"type\":\"ConnectorPlacement.EquallySpacedConnector\",\"uuid\":\"79253ea6-cd7f-4983-840a-f5cee3a4dd91\"}],\"packageUris\":[\"http://schema.mathworks.com/mf0/Connector/R2020b\"],\"version\":\"1.0\"}"
      mask TypeOptions input_type: Drive cycle | Ramp | Step
      mask Callback input_type:
      | activeVariant = get_param(gcb, 'input_type');
      | set_param([gcb '/Inputs'], 'OverrideUsingVariant', activeVariant)
      mask Display:
      | blk = get_param([gcb, '/Inputs'], 'CompiledActiveChoiceBlock');
      | eval(get_param(blk, 'MaskDisplay'))
  Solver Configuration1 : nesl_utility/Solver Configuration  PhysicalDomain=network_engine_domain  SubClassName=solver  LeftPortType=input  RightPortType=generic  Tones=[]  Harmonics=[]  SimulateNoise=off  Profile=off  UseLocalSampling=off  EnableSwitchedLinearOptims=on  FrequencyDomain=off  UseCCode=off  RelTol=0.001  AbsTol=1e-06  MinStep=1e-09  ToWorkspace=off  RevertToSquareIcSolve=off  NumHomotopyIterations=100  PhasorMode=off  PhasorModeNumHarmonics=1  ConsistencySolver=NEWTON_XTOL_AFTER_FTOL  IndexReductionMethod=DerivativeReplacement  DoDC=off  ResidualTolerance=1e-09  ConsistencyTolSource=GLOBAL  ConsistencyAbsTol=0.001  ConsistencyRelTol=0.001  ConsistencyTolFactor=0.001  UseLocalSolver=off  LocalSolverChoice=NE_BACKWARD_EULER_ADVANCER  ResolveIndetEquations=on  FunctionEvalNumThread=1  LocalSolverSampleTime=0.001  DoFixedCost=off  MaxNonlinIter=3  MaxModeIter=2  ComputeImpulses=off  ImpulseIterations=2  LinearAlgebra=auto  LinearAlgebraNumThread=0  EquationFormulation=NE_TIME_EF  DelaysMemoryBudget=1024  AutomaticFiltering=on  FilteringTimeConstant=0.001  PartitionStorageMethod=AS_NEEDED  PartitionMemoryBudget=1024  PartitionMethod=ROBUST
  tag scope: i_dcdc=global, v_dcdc=global
  wires:
  Battery System/1(Batt_Info) -> [Batt_Info]
  Battery System/2(i_dcdc) -> [i_dcdc]
  [Pt] -> Battery System/1(P_Acc)
  Battery System/3(v_dcdc) -> [v_dcdc]
  connections:
  Battery System/RConn1 -- Electrical Load9/RConn1
  Battery System/RConn2 -- Solver Configuration1/RConn1 -- Electrical Load9/RConn2
